simulink model "control_model_gear_position"  (R2015a)
settings: Solver=ode45  StartTime=0  StopTime=1000  FixedStep=0.01  RelTol=1e-3
undefined symbols (not defined in the file): ki, kp
settings Model: SimulationMode=rapid-accelerator  Creator=keysie  LastModifiedBy=keysie
settings DataIOCC: LimitDataPoints=off  SaveFormat=StructureWithTime  SaveOutput=off  SignalLogging=off  SaveTime=off

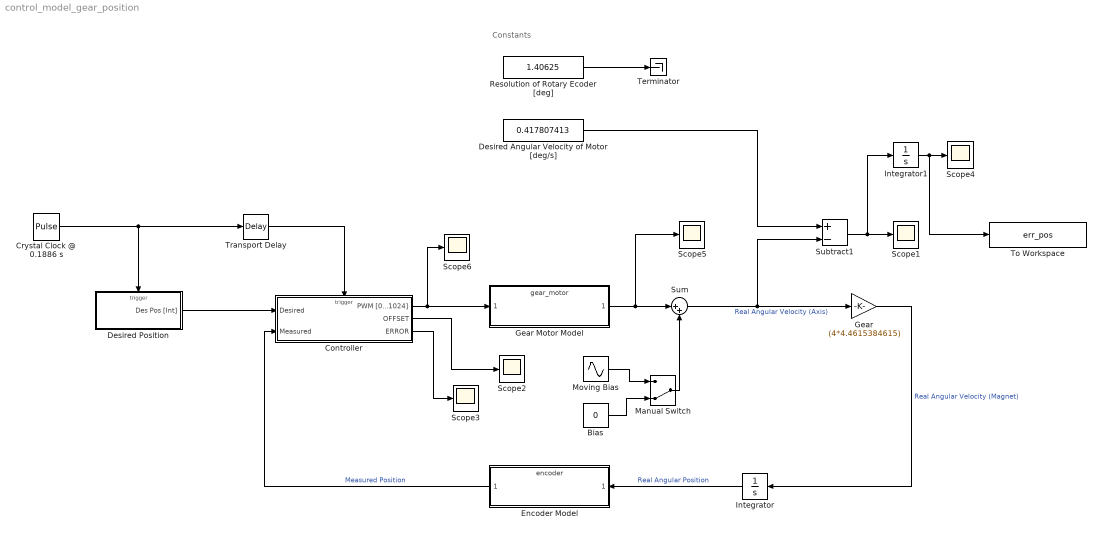
== system control_model_gear_position ==
  note: Constants
  Bias : Constant  Value=0
  Controller : Subsystem  TreatAsAtomicUnit=on
  Crystal Clock @ 0.1886 s : DiscretePulseGenerator  PulseType=Time based  Period=0.188600031806  PulseWidth=5
  Desired Angular Velocity of Motor [deg/s] : Constant  Value=0.417807413
  Desired Position : Subsystem  TreatAsAtomicUnit=on
  Encoder Model : ModelReference  ModelNameDialog=encoder.slx  SimulationMode=Normal  ModelReferenceVersion=1.5  CopyOfModelName=encoder.slx  DefaultDataLogging=on
  Gear : Gain  Gain=(4*4.4615384615)
  Gear Motor Model : ModelReference  ModelNameDialog=gear_motor.slx  SimulationMode=Normal  ModelReferenceVersion=1.24  CopyOfModelName=gear_motor.slx  DefaultDataLogging=on
  Integrator : Integrator
  Integrator1 : Integrator
  Manual Switch : ManualSwitch  CurrentSetting=0
  Moving Bias : Sin  Amplitude=0.2  Frequency=0.2/(2*pi)  SampleTime=0
  Resolution of Rotary Ecoder [deg] : Constant  Value=1.40625
  Scope{1..6} (6 alike) : Scope
      Scope1 settings: TimeRange=300
      Scope2 settings: TimeRange=100  SaveName=ScopeData2
      Scope3 settings: SaveName=ScopeData6
      Scope4 settings: TimeRange=300
      Scope5 settings: TimeRange=300  SaveName=ScopeData3
      Scope6 settings: TimeRange=100  SaveName=ScopeData4
  Subtract1 : Sum  Inputs=+-
  Sum : Sum  Inputs=|++
  Terminator : Terminator
  To Workspace : ToWorkspace  VariableName=err_pos  SampleTime=-1
  Transport Delay : TransportDelay  DelayTime=0.01
  wires:
  Gear Motor Model/1 -> Sum/1, Scope5/1
  Integrator/1 -> Encoder Model/1  "Real Angular Position"
  Encoder Model/1 -> Controller/2(Measured)  "Measured Position"
  Crystal Clock @ 0.1886 s/1 -> Desired Position/Trigger, Transport Delay/1
  Desired Position/1(Des Pos [Int]) -> Controller/1(Desired)
  Controller/1(PWM [0...1024]) -> Scope6/1, Gear Motor Model/1
  Controller/2(OFFSET) -> Scope2/1
  Subtract1/1 -> Integrator1/1, Scope1/1
  Controller/3(ERROR) -> Scope3/1
  Transport Delay/1 -> Controller/Trigger
  Desired Angular Velocity of Motor [deg/s]/1 -> Subtract1/1
  Resolution of Rotary Ecoder [deg]/1 -> Terminator/1
  Sum/1 -> Gear/1, Subtract1/2  "Real Angular Velocity (Axis)"
  Gear/1 -> Integrator/1  "Real Angular Velocity (Magnet)"
  Integrator1/1 -> To Workspace/1, Scope4/1
  Manual Switch/1 -> Sum/2
  Moving Bias/1 -> Manual Switch/1
  Bias/1 -> Manual Switch/2

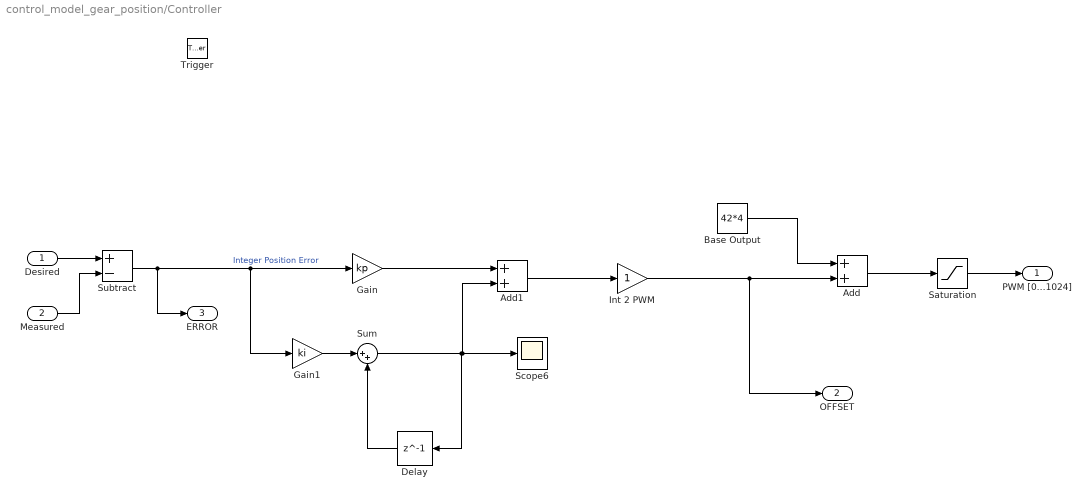
== system control_model_gear_position/Controller ==
  Desired : Inport
  Measured : Inport  Port=2
  Trigger : TriggerPort
  Add : Sum
  Add1 : Sum
  Base Output : Constant  Value=42*4
  Delay : Delay  DelayLength=1
  Gain : Gain  Gain=kp
  Gain1 : Gain  Gain=ki
  Int 2 PWM : Gain
  Saturation : Saturate  UpperLimit=1024  LowerLimit=0
  Scope6 : Scope
      settings: TimeRange=100  SaveName=ScopeData5
  Subtract : Sum  Inputs=+-
  Sum : Sum  Inputs=|++
  PWM [0...1024] : Outport  InitialOutput=[0]
  OFFSET : Outport  Port=2  InitialOutput=[0]
  ERROR : Outport  Port=3  InitialOutput=[0]
  wires:
  Base Output/1 -> Add/1
  Add/1 -> Saturation/1
  Subtract/1 -> ERROR/1, Gain/1, Gain1/1  "Integer Position Error"
  Gain/1 -> Add1/1
  Add1/1 -> Int 2 PWM/1
  Int 2 PWM/1 -> OFFSET/1, Add/2
  Sum/1 -> Scope6/1, Add1/2, Delay/1
  Delay/1 -> Sum/2
  Desired/1 -> Subtract/1
  Measured/1 -> Subtract/2
  Saturation/1 -> PWM [0...1024]/1
  Gain1/1 -> Sum/1

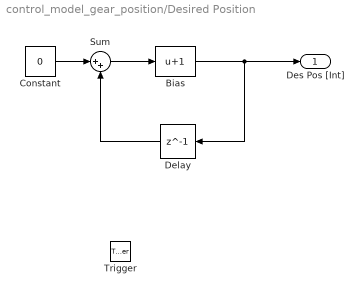
== system control_model_gear_position/Desired Position ==
  Trigger : TriggerPort
  Bias : Bias  Bias=1
  Constant : Constant  Value=0
  Delay : Delay  DelayLength=1
  Sum : Sum  Inputs=|++
  Des Pos [Int] : Outport  InitialOutput=[0]
  wires:
  Bias/1 -> Delay/1, Des Pos [Int]/1
  Delay/1 -> Sum/2
  Constant/1 -> Sum/1
  Sum/1 -> Bias/1
